simulink model "e7g"  (R2021a)
settings: Solver=VariableStepAuto  StartTime=0.0  StopTime=10.0  RelTol=1e-3
undefined symbols (not defined in the file or in its folder): strel
libraries: visionmorphops x4, visionconversions x3, visionsources x1
settings Model: Creator=pranshu  LastModifiedBy=pranshu

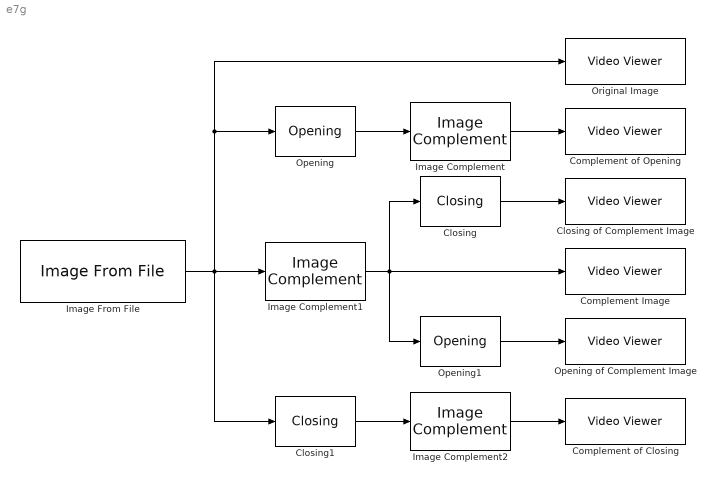
== system e7g ==
  Closing : visionmorphops/Closing  nhoodsrc=Specify via dialog  strel=strel('line',5,45)
      settings: SourceProductBaseCode=VP
  Closing of Complement Image : VideoViewer  FigPos=[578.6 821.2 417.6 304]
  Closing1 : visionmorphops/Closing  nhoodsrc=Specify via dialog  strel=strel('line',5,45)
      settings: SourceProductBaseCode=VP
  Complement Image : VideoViewer  FigPos=[159.4 820.4 417.6 304]
  Complement of Closing : VideoViewer  FigPos=[996.2 409.2 417.6 304]
  Complement of Opening : VideoViewer  FigPos=[577.8 409.2 417.6 304]
  Image Complement : visionconversions/Image Complement
      settings: SourceProductBaseCode=VP
  Image Complement1 : visionconversions/Image Complement
      settings: SourceProductBaseCode=VP
  Image Complement2 : visionconversions/Image Complement
      settings: SourceProductBaseCode=VP
  Image From File : visionsources/Image From File  Tag=vipblks_nd  FileName=coins.png  Ts=inf  imagePorts=One multidimensional signal  OutPortLabels=R|G|B  ImageDataType=Inherit from input image  sdImageDataType=uint(8)  Signed=on  WordLength=16  FractionLengthMode=User-defined  FractionLength=15
  Opening : visionmorphops/Opening  nhoodsrc=Specify via dialog  strel=strel('disk',5)
      settings: SourceProductBaseCode=VP
  Opening of Complement Image : VideoViewer  FigPos=[996.2 820.4 417.6 304]
  Opening1 : visionmorphops/Opening  nhoodsrc=Specify via dialog  strel=strel('disk',5)
      settings: SourceProductBaseCode=VP
  Original Image : VideoViewer  FigPos=[159.4 409.2 417.6 304]
  wires:
  Image From File/1 -> Closing1/1, Opening/1, Original Image/1, Image Complement1/1
  Image Complement/1 -> Complement of Opening/1
  Opening/1 -> Image Complement/1
  Image Complement1/1 -> Opening1/1, Closing/1, Complement Image/1
  Closing/1 -> Closing of Complement Image/1
  Opening1/1 -> Opening of Complement Image/1
  Image Complement2/1 -> Complement of Closing/1
  Closing1/1 -> Image Complement2/1
